simulink model "Q1_Part_c3"  (R2016b)
settings: Solver=ode45  StartTime=0.0  StopTime=14  RelTol=1e-10  AbsTol=1e-10  EnableMultiTasking=on
libraries: cstblocks x2
settings Model: Creator=yarde_000  LastModifiedBy=nadav
settings DataIOCC: LimitDataPoints=on  SaveFormat=Array
settings OptimizationCC: LifeSpan=inf
settings DebuggingCC: SFUnexpectedBacktrackingDiag=warning  SFNoUnconditionalDefaultTransitionDiag=warning  SFExecutionAtInitializationDiag=none
settings HardwareCC: ProdBitPerPointer=32  ProdBitPerSizeT=32  ProdBitPerPtrDiffT=32  ProdLargestAtomicFloat=None  ProdIntDivRoundTo=Undefined  ProdEndianess=Unspecified  ProdWordSize=32  ProdHWDeviceType=32-bit Generic
settings ModelReferenceCC: PropagateSignalLabelsOutOfModel=off
settings GRTTargetCC: TargetLangStandard=C89/C90 (ANSI)  GeneratePreprocessorConditionals=Disable all
settings ConfigComp: CovMetricSettings=dw  CovHtmlReporting=on  CovSaveCumulativeToWorkspaceVar=on  CovSaveSingleToWorkspaceVar=on  CovExternalEMLEnable=off

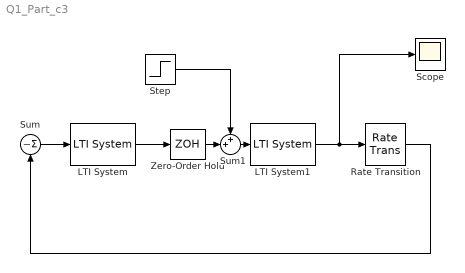
== system Q1_Part_c3 ==
  LTI System : cstblocks/LTI System  sys=Cd_s  IC=[]
  LTI System1 : cstblocks/LTI System  sys=P  IC=[]
  Rate Transition : RateTransition  OutPortSampleTime=ts_s
  Scope : Scope
  Step : Step  Time=0  SampleTime=0
  Sum : Sum  Inputs=||-
  Sum1 : Sum  Inputs=++|
  Zero-Order Hold : ZeroOrderHold  SampleTime=-1
  wires:
  LTI System/1 -> Zero-Order Hold/1
  LTI System1/1 -> Scope/1, Rate Transition/1
  Rate Transition/1 -> Sum/1
  Sum/1 -> LTI System/1
  Zero-Order Hold/1 -> Sum1/2
  Sum1/1 -> LTI System1/1
  Step/1 -> Sum1/1
